simulink model "text28"  (R2014a)
settings: Solver=FixedStepDiscrete  StartTime=0.0  StopTime=10.0  FixedStep=0.0005  RelTol=1e-3
libraries: simulink x70, ec55xxlib x61
(part 1 of 3)
settings Model: Creator=HP  LastModifiedBy=30858
settings OptimizationCC: InlineParams=on  InlineInvariantSignals=on  RollThreshold=9  StateBitsets=on  DataBitsets=on  UseTempVars=on  ZeroExternalMemoryAtStartup=off  ZeroInternalMemoryAtStartup=off  EfficientFloat2IntCast=on  OptimizeModelRefInitCode=on  LifeSpan=1
settings DebuggingCC: InheritedTsInSrcMsg=none
settings HardwareCC: ProdLargestAtomicInteger=Long  ProdLargestAtomicFloat=Double  ProdIntDivRoundTo=Zero  ProdEndianess=BigEndian  ProdHWDeviceType=Freescale MPC5500
settings RTWCC: SystemTargetFile=ec55xx.tlc  MakeCommand=make_rtw optimized_fixed_point=1  GenerateMakefile=off  TemplateMakefile=ec55xx_lcc.tmf  PostCodeGenCommand=ec55xx_pst_s2(buildInfo)  Description=Target for EC55XX  GenerateReport=on  ProcessScript=ec55xx_make_rtw_hook  IncludeHyperlinkInReport=on  LaunchReport=on
settings CodeAppCC: IgnoreCustomStorageClasses=off
settings STFCustomTargetCC: ModelReferenceCompliant=off  ConcurrentExecutionCompliant=off  IncludeMdlTerminateFcn=off  GeneratePreprocessorConditionals=Use local settings  CombineOutputUpdateFcns=on  SuppressErrorStatus=on  ERTCustomFileBanners=on  SupportContinuousTime=off  SupportNonInlinedSFcns=off  MATLABClassNameForMDSCustomization=Simulink.SoftwareTarget.ERTCustomization  GRTInterface=off  SystemTargetFile=ec55xx.tlc
settings ERTTargetCC: GenerateSampleERTMain=off  ModelReferenceCompliant=off  IncludeMdlTerminateFcn=off  SuppressErrorStatus=on  GenerateASAP2=on  ERTSrcFileBannerTemplate=ec55xx_code_template.cgt  ERTHdrFileBannerTemplate=ec55xx_code_template.cgt  ERTDataSrcFileTemplate=ec55xx_code_template.cgt  ERTDataHdrFileTemplate=ec55xx_code_template.cgt  ERTCustomFileTemplate=ec55xx_file_process.tlc

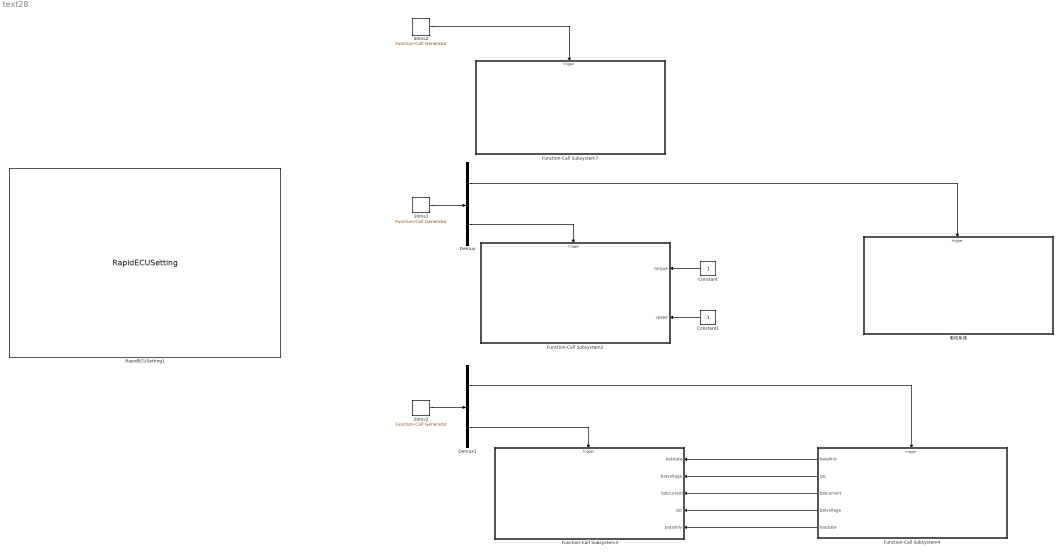
== system text28 ==
  10ms1 : simulink/Ports & Subsystems/Function-Call Generator  sample_time=0.01  numberOfIterations=1
  20ms2 : simulink/Ports & Subsystems/Function-Call Generator  sample_time=0.2  numberOfIterations=1
  50ms2 : simulink/Ports & Subsystems/Function-Call Generator  sample_time=0.05  numberOfIterations=1
  Constant : Constant
  Constant1 : Constant
  Demux : Demux  Outputs=2
  Demux1 : Demux  Outputs=2
  Function-Call Subsystem2 : Subsystem  TreatAsAtomicUnit=on
  Function-Call Subsystem3 : Subsystem  TreatAsAtomicUnit=on
  Function-Call Subsystem4 : Subsystem  TreatAsAtomicUnit=on
  Function-Call Subsystem7 : Subsystem  TreatAsAtomicUnit=on
  RapidECUSetting1 : ec55xxlib/RapidECU_U2/RapidECUSetting
      link override CAN: apdf=1  acmt=Extended(29-bit ID)  bcmt=Extended(29-bit ID)  ccmt=Standard(11-bit ID)
      link override CCP: idtype=Extended(29-bit ID)
      link override CPU: wdgenable=on  counter=104ms
      link override RTI: rtiperiod=0.0005
  驱动系统 : Subsystem  TreatAsAtomicUnit=on
  wires:
  10ms1/1 -> Demux/1
  20ms2/1 -> Demux1/1
  50ms2/1 -> Function-Call Subsystem7/Trigger
  Demux/1 -> 驱动系统/Trigger
  Demux/2 -> Function-Call Subsystem2/Trigger
  Demux1/1 -> Function-Call Subsystem4/Trigger
  Demux1/2 -> Function-Call Subsystem3/Trigger
  Function-Call Subsystem4/1(batalmlv) -> Function-Call Subsystem3/1(batstate)
  Function-Call Subsystem4/2(soc) -> Function-Call Subsystem3/2(batvoltage)
  Function-Call Subsystem4/3(batcurrent) -> Function-Call Subsystem3/3(batcurrent)
  Function-Call Subsystem4/4(batvoltage) -> Function-Call Subsystem3/4(soc)
  Function-Call Subsystem4/5(batstate) -> Function-Call Subsystem3/5(batalmlv)
  Constant/1 -> Function-Call Subsystem2/1(torque)
  Constant1/1 -> Function-Call Subsystem2/2(speed)

== system text28/Function-Call Subsystem2 ==
  torque : Inport
  speed : Inport  Port=2
  function : TriggerPort  TriggerType=function-call
  CANTransmit : ec55xxlib/RapidECU_U2/07CANCommucation/CANTransmit  canmodule=A  canbuffer=8  canmessageid=hex2dec('3E4')  canmessagetype=Standard(11-bit ID)  datalength=8  sampletime=-1
  xieyi : Subsystem
  xieyi_Ter : Terminator
  wires:
  CANTransmit/1 -> xieyi_Ter/1
  xieyi/1(output) -> CANTransmit/1
  speed/1 -> xieyi/1(Speed_in)
  torque/1 -> xieyi/2(Motor_toque_in)

== system text28/Function-Call Subsystem3 ==
  batstate : Inport
  batvoltage : Inport  Port=2
  batcurrent : Inport  Port=3
  soc : Inport  Port=4
  batalmlv : Inport  Port=5
  function : TriggerPort  TriggerType=function-call
  CANTransmit : ec55xxlib/RapidECU_U2/07CANCommucation/CANTransmit  canmodule=A  canbuffer=8  canmessageid=hex2dec('015')  canmessagetype=Standard(11-bit ID)  datalength=8  sampletime=-1
  dianchi : Subsystem
  dianchi_Ter : Terminator
  wires:
  CANTransmit/1 -> dianchi_Ter/1
  dianchi/1(output) -> CANTransmit/1
  batvoltage/1 -> dianchi/3(BatVoltage_in)
  batstate/1 -> dianchi/1(BatState_in)
  batalmlv/1 -> dianchi/2(BatAlmLv_in)
  soc/1 -> dianchi/4(BatSoc_in)
  batcurrent/1 -> dianchi/5(BatCurrent_in)

== system text28/Function-Call Subsystem4 ==
  function : TriggerPort  TriggerType=function-call
  CAN检测 : ec55xxlib/RapidECU_U2/07CANCommucation/CANReceive  canmodule=A  canbuffer=0  canmessageid=hex2dec('186040F3')  canmessagetype=Extended(29-bit ID)  datalength=8  sampletime=-1
  Function-Call Subsystem4 : Subsystem  TreatAsAtomicUnit=on
  Logical Operator : Logic  Inputs=3  AllPortsSameDT=off  OutDataTypeStr=boolean
  MeaModule2 : ec55xxlib/RapidECU_U2/11Calibration/MeaModule  signal=bms_sign
  MeaModule5 : ec55xxlib/RapidECU_U2/11Calibration/MeaModule  signal=bms_canok
  ReceiveMessages : Subsystem
  Terminator : Terminator
  Terminator1 : Terminator
  Terminator3 : Terminator
  "can断线 " : Subsystem
  一级警告 : Subsystem
  可视 : Subsystem
  故障状态报警 : Subsystem
  batalmlv : Outport
  soc : Outport  Port=2
  batcurrent : Outport  Port=3
  batvoltage : Outport  Port=4
  batstate : Outport  Port=5
  wires:
  CAN检测/1 -> Function-Call Subsystem4/Trigger
  CAN检测/5 -> Terminator1/1
  CAN检测/4 -> Function-Call Subsystem4/2(In3)
  MeaModule5/1 -> Function-Call Subsystem4/1(1n1)
  CAN检测/3 -> Terminator3/1
  ReceiveMessages/1(batstate) -> 故障状态报警/1(In1), batstate/1
  Logical Operator/1 -> MeaModule2/1
  一级警告/1(Out1) -> Logical Operator/2
  故障状态报警/1(Out1) -> Logical Operator/1
  CAN检测/2 -> "can断线 "/1(In1), MeaModule5/1
  Function-Call Subsystem4/1(Out1) -> ReceiveMessages/1(In1)
  ReceiveMessages/2("batalmlv ") -> 一级警告/1(In1), batalmlv/1
  ReceiveMessages/3(soc) -> soc/1
  ReceiveMessages/4(batcurrent) -> batcurrent/1
  ReceiveMessages/5(batvoltage) -> batvoltage/1
  "can断线 "/1(Out1) -> Logical Operator/3
  MeaModule2/1 -> Terminator/1

== system text28/Function-Call Subsystem7 ==
  function : TriggerPort  TriggerType=function-call
  Constant1 : Constant  Value=50
  Constant2 : Constant  Value=50
  Constant3 : Constant
  Data Type Conversion1 : DataTypeConversion  OutDataTypeStr=uint32
  Data Type Conversion2 : DataTypeConversion  OutDataTypeStr=uint32
  Function-Call Subsystem2 : Subsystem  TreatAsAtomicUnit=on
  Logical Operator : Logic  Operator=OR  AllPortsSameDT=off  OutDataTypeStr=boolean
  MCU STATUS 2 : ec55xxlib/RapidECU_U2/07CANCommucation/CANReceive  canmodule=B  canbuffer=0  canmessageid=hex2dec('CFF0109 ')  canmessagetype=Extended(29-bit ID)  datalength=8  sampletime=-1
  MCU_STATUS_2 : Subsystem
  MeaModule : ec55xxlib/RapidECU_U1/11Calibration/MeaModule  signal=FAN_sign
  PowerDriverPWM : ec55xxlib/RapidECU_U2/06PowerDriverPWM/PowerDriverPWM  channel=118: O_PWM12_HS2A9  sampletime=-1
  Relational Operator : RelationalOperator  OutDataTypeStr=boolean
  Relational Operator1 : RelationalOperator  OutDataTypeStr=boolean
  Terminator2 : Terminator
  Terminator4 : Terminator
  Terminator5 : Terminator
  wires:
  MCU STATUS 2/1 -> Function-Call Subsystem2/Trigger
  MCU STATUS 2/3 -> Terminator2/1
  MCU STATUS 2/5 -> Terminator4/1
  MCU STATUS 2/2 -> Terminator5/1
  Function-Call Subsystem2/1(out1) -> MCU_STATUS_2/1(In1)
  MCU STATUS 2/4 -> Function-Call Subsystem2/1(In1)
  MCU_STATUS_2/1(Motor_Tem) -> Relational Operator/1
  MCU_STATUS_2/2(MCU_Tem) -> Relational Operator1/1
  Relational Operator/1 -> Logical Operator/1
  Relational Operator1/1 -> Logical Operator/2
  Constant1/1 -> Relational Operator1/2
  Constant2/1 -> Relational Operator/2
  Data Type Conversion1/1 -> PowerDriverPWM/2
  Constant3/1 -> Data Type Conversion2/1
  Data Type Conversion2/1 -> PowerDriverPWM/1
  Logical Operator/1 -> MeaModule/1
  MeaModule/1 -> Data Type Conversion1/1

== system text28/驱动系统 ==
  function : TriggerPort  TriggerType=function-call
  Constant : Constant
  Data Type Conversion : DataTypeConversion  OutDataTypeStr=boolean
  ECU : Subsystem
  MCU_CAN发送 : Subsystem
  MainRelaySwitch : ec55xxlib/RapidECU_U2/09PowerManagement/MainRelaySwitch  sampletime=-1
  WDGFeed : ec55xxlib/RapidECU_U2/08MCUManagement/WDGFeed  sampletime=-1
  安全回路输出 : Subsystem
  驱动逻辑 : Subsystem
  wires:
  ECU/1(Out1) -> MCU_CAN发送/1(In1)
  Data Type Conversion/1 -> MainRelaySwitch/1
  驱动逻辑/2(复位) -> ECU/2(保留)
  驱动逻辑/1(油门输出) -> ECU/1(扭矩请求)
  Constant/1 -> Data Type Conversion/1
  MCU_CAN发送/1(系统关键信号) -> 安全回路输出/1(In1)
  驱动逻辑/4(系统关键信号) -> 安全回路输出/2(In2)
  驱动逻辑/3(使能) -> ECU/3(使能)
  ? -> ?
  ? -> ?
  ? -> ?
  ? -> ?

== system text28/Function-Call Subsystem2/xieyi ==
  Speed_in : Inport
  Motor_toque_in : Inport  Port=2
  Conv{1..8} (8 alike) : DataTypeConversion
  Motor_toque : Subsystem
  Speed : Subsystem
  or{1..8} (8 alike) : simulink/Logic and Bit Operations/Bitwise Operator  logicop=OR  UseBitMask=off  NumInputPorts=2  BitMask=bin2dec('11011001')  BitMaskRealWorld=Stored Integer
  xieyi_DLC : Constant  Value=2  OutDataTypeStr=uint8
  xieyi_DLC_Out : Terminator
  xieyi_ID : Constant  Value=995  OutDataTypeStr=single
  xieyi_ID_Out : Terminator
  xieyi_mux : Mux  Inputs=8
  output : Outport
  wires:
  xieyi_mux/1 -> output/1
  Speed/1(output1) -> or1/1
  Speed/2(output2) -> or2/1
  Speed/3(output3) -> or3/1
  Speed/4(output4) -> or4/1
  Speed/5(output5) -> or5/1
  Speed/6(output6) -> or6/1
  Speed/7(output7) -> or7/1
  Speed/8(output8) -> or8/1
  Motor_toque/1(output1) -> or1/2
  Motor_toque/2(output2) -> or2/2
  Motor_toque/3(output3) -> or3/2
  Motor_toque/4(output4) -> or4/2
  Motor_toque/5(output5) -> or5/2
  Motor_toque/6(output6) -> or6/2
  Motor_toque/7(output7) -> or7/2
  Motor_toque/8(output8) -> or8/2
  or1/1 -> Conv1/1
  Conv1/1 -> xieyi_mux/1
  or2/1 -> Conv2/1
  Conv2/1 -> xieyi_mux/2
  or3/1 -> Conv3/1
  Conv3/1 -> xieyi_mux/3
  or4/1 -> Conv4/1
  Conv4/1 -> xieyi_mux/4
  or5/1 -> Conv5/1
  Conv5/1 -> xieyi_mux/5
  or6/1 -> Conv6/1
  Conv6/1 -> xieyi_mux/6
  or7/1 -> Conv7/1
  Conv7/1 -> xieyi_mux/7
  or8/1 -> Conv8/1
  Conv8/1 -> xieyi_mux/8
  xieyi_ID/1 -> xieyi_ID_Out/1
  xieyi_DLC/1 -> xieyi_DLC_Out/1
  Speed_in/1 -> Speed/1(Speed)
  Motor_toque_in/1 -> Motor_toque/1(Motor_toque)

== system text28/Function-Call Subsystem3/dianchi ==
  BatState_in : Inport
  BatAlmLv_in : Inport  Port=2
  BatVoltage_in : Inport  Port=3
  BatSoc_in : Inport  Port=4
  BatCurrent_in : Inport  Port=5
  BatAlmLv : Subsystem
  BatCurrent : Subsystem
  BatSoc : Subsystem
  BatState : Subsystem
  BatVoltage : Subsystem
  Conv{1..8} (8 alike) : DataTypeConversion
  dianchi_DLC : Constant  Value=7  OutDataTypeStr=uint8
  dianchi_DLC_Out : Terminator
  dianchi_ID : Constant  Value=2556444915  OutDataTypeStr=single
  dianchi_ID_Out : Terminator
  dianchi_mux : Mux  Inputs=8
  or{1..8} (8 alike) : simulink/Logic and Bit Operations/Bitwise Operator  logicop=OR  UseBitMask=off  NumInputPorts=5  BitMask=bin2dec('11011001')  BitMaskRealWorld=Stored Integer
  output : Outport
  wires:
  dianchi_mux/1 -> output/1
  BatState/1(output1) -> or1/1
  BatState/2(output2) -> or2/1
  BatState/3(output3) -> or3/1
  BatState/4(output4) -> or4/1
  BatState/5(output5) -> or5/1
  BatState/6(output6) -> or6/1
  BatState/7(output7) -> or7/1
  BatState/8(output8) -> or8/1
  BatAlmLv/1(output1) -> or1/2
  BatAlmLv/2(output2) -> or2/2
  BatAlmLv/3(output3) -> or3/2
  BatAlmLv/4(output4) -> or4/2
  BatAlmLv/5(output5) -> or5/2
  BatAlmLv/6(output6) -> or6/2
  BatAlmLv/7(output7) -> or7/2
  BatAlmLv/8(output8) -> or8/2
  BatVoltage/1(output1) -> or1/3
  BatVoltage/2(output2) -> or2/3
  BatVoltage/3(output3) -> or3/3
  BatVoltage/4(output4) -> or4/3
  BatVoltage/5(output5) -> or5/3
  BatVoltage/6(output6) -> or6/3
  BatVoltage/7(output7) -> or7/3
  BatVoltage/8(output8) -> or8/3
  BatSoc/1(output1) -> or1/4
  BatSoc/2(output2) -> or2/4
  BatSoc/3(output3) -> or3/4
  BatSoc/4(output4) -> or4/4
  BatSoc/5(output5) -> or5/4
  BatSoc/6(output6) -> or6/4
  BatSoc/7(output7) -> or7/4
  BatSoc/8(output8) -> or8/4
  BatCurrent/1(output1) -> or1/5
  BatCurrent/2(output2) -> or2/5
  BatCurrent/3(output3) -> or3/5
  BatCurrent/4(output4) -> or4/5
  BatCurrent/5(output5) -> or5/5
  BatCurrent/6(output6) -> or6/5
  BatCurrent/7(output7) -> or7/5
  BatCurrent/8(output8) -> or8/5
  or1/1 -> Conv1/1
  Conv1/1 -> dianchi_mux/1
  or2/1 -> Conv2/1
  Conv2/1 -> dianchi_mux/2
  or3/1 -> Conv3/1
  Conv3/1 -> dianchi_mux/3
  or4/1 -> Conv4/1
  Conv4/1 -> dianchi_mux/4
  or5/1 -> Conv5/1
  Conv5/1 -> dianchi_mux/5
  or6/1 -> Conv6/1
  Conv6/1 -> dianchi_mux/6
  or7/1 -> Conv7/1
  Conv7/1 -> dianchi_mux/7
  or8/1 -> Conv8/1
  Conv8/1 -> dianchi_mux/8
  dianchi_ID/1 -> dianchi_ID_Out/1
  dianchi_DLC/1 -> dianchi_DLC_Out/1
  BatState_in/1 -> BatState/1(BatState)
  BatAlmLv_in/1 -> BatAlmLv/1(BatAlmLv)
  BatVoltage_in/1 -> BatVoltage/1(BatVoltage)
  BatSoc_in/1 -> BatSoc/1(BatSoc)
  BatCurrent_in/1 -> BatCurrent/1(BatCurrent)

== system text28/Function-Call Subsystem4/Function-Call Subsystem4 ==
  1n1 : Inport
  In3 : Inport  Port=2
  function : TriggerPort  TriggerType=function-call
  Terminator2 : Terminator
  Out1 : Outport
  wires:
  1n1/1 -> Terminator2/1
  In3/1 -> Out1/1

== system text28/Function-Call Subsystem4/ReceiveMessages ==
  In1 : Inport
  BMS_HCU_INFO : Subsystem
  BatLife_Ter : Terminator
  BtaSOH_Ter : Terminator
  MeaModule : ec55xxlib/RapidECU_U2/11Calibration/MeaModule  signal=baojing
  MeaModule1 : ec55xxlib/RapidECU_U2/11Calibration/MeaModule  signal=soc
  MeaModule2 : ec55xxlib/RapidECU_U2/11Calibration/MeaModule  signal=zhuangtai
  MeaModule3 : ec55xxlib/RapidECU_U2/11Calibration/MeaModule  signal=dianya
  batstate : Outport
  "batalmlv " : Outport  Port=2
  soc : Outport  Port=3
  batcurrent : Outport  Port=4
  batvoltage : Outport  Port=5
  wires:
  BMS_HCU_INFO/1(BtaSOH_Out) -> BtaSOH_Ter/1
  BMS_HCU_INFO/5(BatLife_Out) -> BatLife_Ter/1
  BMS_HCU_INFO/6(BatCurrent_Out) -> batcurrent/1
  In1/1 -> BMS_HCU_INFO/1(input)
  BMS_HCU_INFO/7(BatAlmLv_Out) -> MeaModule/1
  MeaModule/1 -> "batalmlv "/1
  BMS_HCU_INFO/4(BatSoc_Out) -> MeaModule1/1
  MeaModule1/1 -> soc/1
  BMS_HCU_INFO/3(BatState_Out) -> MeaModule2/1
  MeaModule2/1 -> batstate/1
  BMS_HCU_INFO/2(BatVoltage_Out) -> MeaModule3/1
  MeaModule3/1 -> batvoltage/1

== system text28/Function-Call Subsystem4/can断线  ==
  In1 : Inport
  If Action Subsystem2 : Subsystem  TreatAsAtomicUnit=on
  If Action Subsystem3 : Subsystem  TreatAsAtomicUnit=on
  If1 : If  IfExpression=u1<1
  MeaModule1 : ec55xxlib/RapidECU_U2/11Calibration/MeaModule  signal=bms_sign1
  Merge1 : Merge
  Out1 : Outport
  wires:
  If1/1 -> If Action Subsystem2/Action
  If Action Subsystem2/1(Out1) -> Merge1/1
  MeaModule1/1 -> Out1/1
  If1/2 -> If Action Subsystem3/Action
  If Action Subsystem3/1(Out1) -> Merge1/2
  Merge1/1 -> MeaModule1/1
  In1/1 -> If1/1

== system text28/Function-Call Subsystem4/一级警告 ==
  In1 : Inport
  If : If  IfExpression=u1==1
  If Action Subsystem : Subsystem  TreatAsAtomicUnit=on
  If Action Subsystem1 : Subsystem  TreatAsAtomicUnit=on
  Merge : Merge
  Out1 : Outport
  wires:
  If/1 -> If Action Subsystem/Action
  If/2 -> If Action Subsystem1/Action
  In1/1 -> If/1
  If Action Subsystem/1(Out1) -> Merge/1
  If Action Subsystem1/1(Out1) -> Merge/2
  Merge/1 -> Out1/1

== system text28/Function-Call Subsystem4/可视 ==
  Add : Sum  OutDataTypeStr=uint32
  Constant1 : Constant  OutDataTypeStr=uint32
  Constant4 : Constant  OutDataTypeStr=uint32  SampleTime=-1
  Constant5 : Constant  Value=0  OutDataTypeStr=uint32  SampleTime=-1
  Constant6 : Constant
  Data Type Conversion4 : DataTypeConversion
  Data Type Conversion5 : DataTypeConversion  OutDataTypeStr=uint32
  Display : Display
  Display1 : Display
  MeaModule3 : ec55xxlib/RapidECU_U2/11Calibration/MeaModule  signal=keshi
  Switch : Switch  Criteria=u2 > Threshold  Threshold=5
  Unit Delay : UnitDelay  SampleTime=-1
  断can线亮灯3 : ec55xxlib/RapidECU_U2/06PowerDriverPWM/PowerDriverPWM  channel=58: O_PWM1_LS1A8  sampletime=-1
  wires:
  Data Type Conversion5/1 -> 断can线亮灯3/1
  Data Type Conversion4/1 -> 断can线亮灯3/2
  MeaModule3/1 -> Display/1, Data Type Conversion4/1
  Constant6/1 -> Data Type Conversion5/1
  Constant1/1 -> Add/1
  Constant4/1 -> Switch/1
  Switch/1 -> MeaModule3/1
  Add/1 -> Unit Delay/1, Display1/1, Switch/2
  Unit Delay/1 -> Add/2
  Constant5/1 -> Switch/3

== system text28/Function-Call Subsystem4/故障状态报警 ==
  In1 : Inport
  If : If  IfExpression=u1==7
  If Action Subsystem : Subsystem  TreatAsAtomicUnit=on
  If Action Subsystem1 : Subsystem  TreatAsAtomicUnit=on
  Merge : Merge
  Out1 : Outport
  wires:
  If/1 -> If Action Subsystem/Action
  If/2 -> If Action Subsystem1/Action
  In1/1 -> If/1
  If Action Subsystem/1(Out1) -> Merge/1
  If Action Subsystem1/1(Out1) -> Merge/2
  Merge/1 -> Out1/1

== system text28/Function-Call Subsystem7/Function-Call Subsystem2 ==
  In1 : Inport
  function : TriggerPort  TriggerType=function-call
  out1 : Outport
  wires:
  In1/1 -> out1/1

== system text28/Function-Call Subsystem7/MCU_STATUS_2 ==
  In1 : Inport
  Fail_Grade_out : Terminator
  Live_counter_Ter : Terminator
  MCU_STATUS_2 : Subsystem
  MeaModule5 : ec55xxlib/RapidECU_U1/11Calibration/MeaModule  signal=MotorTemp
  MeaModule6 : ec55xxlib/RapidECU_U1/11Calibration/MeaModule  signal=McuTemp
  Torque_Limit_High_Ter : Terminator
  Torque_Limit_Low_Ter : Terminator
  Motor_Tem : Outport
  MCU_Tem : Outport  Port=2
  wires:
  MCU_STATUS_2/1(Torque_Limit_Low_Out) -> Torque_Limit_Low_Ter/1
  MCU_STATUS_2/2(Torque_Limit_High_Out) -> Torque_Limit_High_Ter/1
  MCU_STATUS_2/5(Live_counter_Out) -> Live_counter_Ter/1
  MCU_STATUS_2/6(Fail_Grade_Out) -> Fail_Grade_out/1
  In1/1 -> MCU_STATUS_2/1(input)
  MeaModule5/1 -> Motor_Tem/1
  MCU_STATUS_2/3(Motor_Temperature_Out) -> MeaModule5/1
  MeaModule6/1 -> MCU_Tem/1
  MCU_STATUS_2/4(MCU_temperature_Out) -> MeaModule6/1

== system text28/驱动系统/ECU ==
  扭矩请求 : Inport
  保留 : Inport  Port=2
  使能 : Inport  Port=3
  Constant : Constant  Value=2
  Constant1 : Constant
  Constant2 : Constant  Value=9000
  FootBrake : Ground
  demand_speed : Ground
  handBrake : Ground
  电机报文打包 : Subsystem
  Out1 : Outport
  wires:
  Constant/1 -> 电机报文打包/8(Control_Mode_in)
  FootBrake/1 -> 电机报文打包/6(FootBrake_in)
  handBrake/1 -> 电机报文打包/5(handBrake_in)
  电机报文打包/1(output) -> Out1/1
  Constant1/1 -> 电机报文打包/7(Gear_in)
  保留/1 -> 电机报文打包/9(Fault_Reset_in)
  使能/1 -> 电机报文打包/10(MCU_Enable_in)
  demand_speed/1 -> 电机报文打包/1(Demand_Speed_in)
  Constant2/1 -> 电机报文打包/4(High_Value_in), 电机报文打包/3(Low_Value_in)
  扭矩请求/1 -> 电机报文打包/2(Demand_Torquee_in)

== system text28/驱动系统/MCU_CAN发送 ==
  In1 : Inport
  CANTransmit : ec55xxlib/RapidECU_U2/07CANCommucation/CANTransmit  canmodule=B  canbuffer=8  canmessageid=hex2dec('CFF09EF')  canmessagetype=Extended(29-bit ID)  datalength=8  sampletime=-1
  MeaModule : ec55xxlib/RapidECU_U2/11Calibration/MeaModule  signal=CAN_ok
  Terminator : Terminator
  安全回路out : Subsystem
  系统关键信号 : Outport
  wires:
  CANTransmit/1 -> MeaModule/1
  In1/1 -> CANTransmit/1
  MeaModule/1 -> 安全回路out/1(CAN ok), Terminator/1
  安全回路out/1(Out1) -> 系统关键信号/1

== system text28/驱动系统/安全回路输出 ==
  In1 : Inport
  In2 : Inport  Port=2
  Constant4 : Constant  OutDataTypeStr=uint32
  Data Type Conversion2 : DataTypeConversion  OutDataTypeStr=uint32
  Logical Operator : Logic  AllPortsSameDT=off  OutDataTypeStr=boolean
  MeaModule1 : ec55xxlib/RapidECU_U2/11Calibration/MeaModule  signal=anquan_out
  安全出 : ec55xxlib/RapidECU_U2/06PowerDriverPWM/PowerDriverPWM  channel=114: O_PWM9_HS2A9  sampletime=-1
  wires:
  Data Type Conversion2/1 -> MeaModule1/1
  Constant4/1 -> 安全出/1
  MeaModule1/1 -> 安全出/2
  Logical Operator/1 -> Data Type Conversion2/1
  In1/1 -> Logical Operator/1
  In2/1 -> Logical Operator/2

== system text28/驱动系统/驱动逻辑 ==
  Drive_AEKF : Subsystem
  制动与尾灯 : Subsystem  TreatAsAtomicUnit=on
  制动与待驶 : Subsystem
  油门规则 : Subsystem
  电机测速 : Subsystem
  角度传感器 : Subsystem
  油门输出 : Outport
  复位 : Outport  Port=2
  使能 : Outport  Port=3
  系统关键信号 : Outport  Port=4
  wires:
  制动与待驶/2(EN) -> 使能/1
  制动与待驶/1(RES) -> 复位/1
  角度传感器/3(系统关键信号判断) -> 系统关键信号/1
  角度传感器/1("油门数值 ") -> 油门规则/1(油门原始值)
  角度传感器/2(油门百分比) -> 油门规则/2(油门百分比)
  电机测速/2(电机扭矩) -> Drive_AEKF/3(Te_raw)
  电机测速/1(电机转速) -> Drive_AEKF/2(w_rpm)
  制动与尾灯/1(油压2) -> 油门规则/3(刹车有效)
  制动与尾灯/2(油压1) -> 制动与待驶/1("制动 ")
  油门规则/1(油门请求) -> Drive_AEKF/1(T_base)
  Drive_AEKF/1(T_opt) -> 油门输出/1

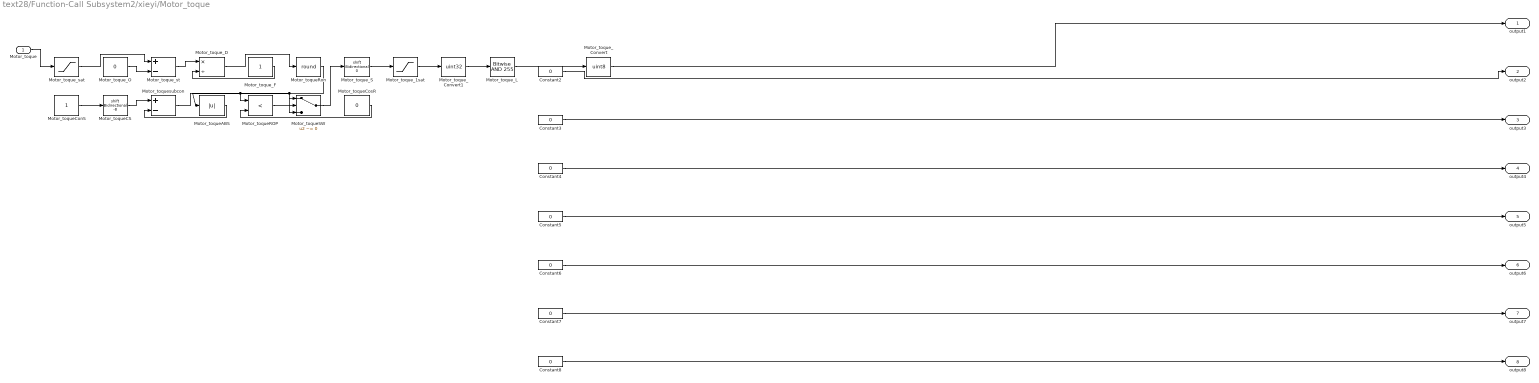
== system text28/Function-Call Subsystem2/xieyi/Motor_toque ==
  Motor_toque : Inport
  Constant{2..8} (7 alike) : Constant  Value=0  OutDataTypeStr=uint8  SampleTime=-1
  Motor_toqueABS : Abs
  Motor_toqueCS : ArithShift  BitShiftNumber=-8
  Motor_toqueConS : Constant  OutDataTypeStr=single
  Motor_toqueCosR : Constant  Value=0  OutDataTypeStr=uint8
  Motor_toqueROP : RelationalOperator  Operator=<  OutDataTypeStr=boolean
  Motor_toqueRon : Rounding  Operator=round
  Motor_toqueSW : Switch  Criteria=u2 ~= 0
  Motor_toque_1sat : Saturate  UpperLimit=255  LowerLimit=0
  Motor_toque_Convert : DataTypeConversion  OutDataTypeStr=uint8
  Motor_toque_Convert1 : DataTypeConversion  OutDataTypeStr=uint32
  Motor_toque_D : Product  Inputs=*/
  Motor_toque_F : Constant  OutDataTypeStr=single
  Motor_toque_L : simulink/Logic and Bit Operations/Bitwise Operator  logicop=AND  UseBitMask=on  BitMask=255  BitMaskRealWorld=Stored Integer
  Motor_toque_O : Constant  Value=0  OutDataTypeStr=single
  Motor_toque_S : ArithShift
  Motor_toque_sat : Saturate  UpperLimit=150  LowerLimit=0
  Motor_toque_st : Sum  Inputs=+-
  Motor_toquesubcon : Sum  Inputs=+-
  output1 : Outport
  output2 : Outport  Port=2
  output3 : Outport  Port=3
  output4 : Outport  Port=4
  output5 : Outport  Port=5
  output6 : Outport  Port=6
  output7 : Outport  Port=7
  output8 : Outport  Port=8
  wires:
  Motor_toque/1 -> Motor_toque_sat/1
  Motor_toque_sat/1 -> Motor_toque_st/1
  Motor_toque_O/1 -> Motor_toque_st/2
  Motor_toque_st/1 -> Motor_toque_D/1
  Motor_toque_F/1 -> Motor_toque_D/2
  Motor_toque_D/1 -> Motor_toqueRon/1
  Motor_toqueRon/1 -> Motor_toqueROP/1, Motor_toqueABS/1, Motor_toqueSW/3
  Motor_toqueCosR/1 -> Motor_toqueROP/2
  Motor_toqueConS/1 -> Motor_toqueCS/1
  Motor_toqueCS/1 -> Motor_toquesubcon/1
  Motor_toqueABS/1 -> Motor_toquesubcon/2
  Motor_toquesubcon/1 -> Motor_toqueSW/1
  Motor_toqueROP/1 -> Motor_toqueSW/2
  Motor_toqueSW/1 -> Motor_toque_S/1
  Motor_toque_S/1 -> Motor_toque_1sat/1
  Motor_toque_1sat/1 -> Motor_toque_Convert1/1
  Motor_toque_Convert1/1 -> Motor_toque_L/1
  Motor_toque_L/1 -> Motor_toque_Convert/1
  Motor_toque_Convert/1 -> output1/1
  Constant2/1 -> output2/1
  Constant3/1 -> output3/1
  Constant4/1 -> output4/1
  Constant5/1 -> output5/1
  Constant6/1 -> output6/1
  Constant7/1 -> output7/1
  Constant8/1 -> output8/1

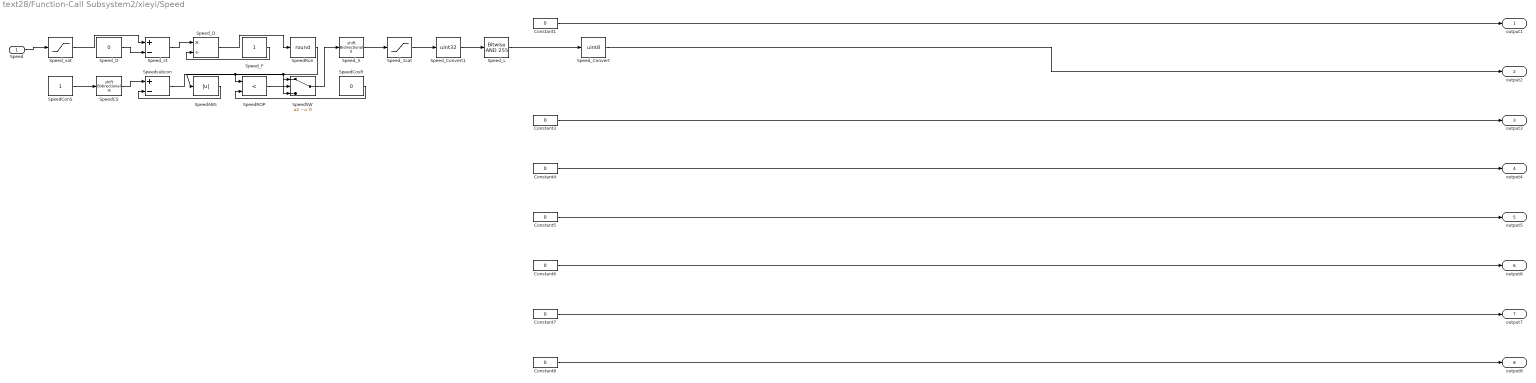
== system text28/Function-Call Subsystem2/xieyi/Speed ==
  Speed : Inport
  Constant{1,3..8} (7 alike) : Constant  Value=0  OutDataTypeStr=uint8  SampleTime=-1
  SpeedABS : Abs
  SpeedCS : ArithShift  BitShiftNumber=-8
  SpeedConS : Constant  OutDataTypeStr=single
  SpeedCosR : Constant  Value=0  OutDataTypeStr=uint8
  SpeedROP : RelationalOperator  Operator=<  OutDataTypeStr=boolean
  SpeedRon : Rounding  Operator=round
  SpeedSW : Switch  Criteria=u2 ~= 0
  Speed_1sat : Saturate  UpperLimit=255  LowerLimit=0
  Speed_Convert : DataTypeConversion  OutDataTypeStr=uint8
  Speed_Convert1 : DataTypeConversion  OutDataTypeStr=uint32
  Speed_D : Product  Inputs=*/
  Speed_F : Constant  OutDataTypeStr=single
  Speed_L : simulink/Logic and Bit Operations/Bitwise Operator  logicop=AND  UseBitMask=on  BitMask=255  BitMaskRealWorld=Stored Integer
  Speed_O : Constant  Value=0  OutDataTypeStr=single
  Speed_S : ArithShift
  Speed_sat : Saturate  UpperLimit=150  LowerLimit=0
  Speed_st : Sum  Inputs=+-
  Speedsubcon : Sum  Inputs=+-
  output1 : Outport
  output2 : Outport  Port=2
  output3 : Outport  Port=3
  output4 : Outport  Port=4
  output5 : Outport  Port=5
  output6 : Outport  Port=6
  output7 : Outport  Port=7
  output8 : Outport  Port=8
  wires:
  Speed/1 -> Speed_sat/1
  Speed_sat/1 -> Speed_st/1
  Speed_O/1 -> Speed_st/2
  Speed_st/1 -> Speed_D/1
  Speed_F/1 -> Speed_D/2
  Speed_D/1 -> SpeedRon/1
  SpeedRon/1 -> SpeedROP/1, SpeedABS/1, SpeedSW/3
  SpeedCosR/1 -> SpeedROP/2
  SpeedConS/1 -> SpeedCS/1
  SpeedCS/1 -> Speedsubcon/1
  SpeedABS/1 -> Speedsubcon/2
  Speedsubcon/1 -> SpeedSW/1
  SpeedROP/1 -> SpeedSW/2
  SpeedSW/1 -> Speed_S/1
  Speed_S/1 -> Speed_1sat/1
  Speed_1sat/1 -> Speed_Convert1/1
  Speed_Convert1/1 -> Speed_L/1
  Speed_L/1 -> Speed_Convert/1
  Speed_Convert/1 -> output2/1
  Constant1/1 -> output1/1
  Constant3/1 -> output3/1
  Constant4/1 -> output4/1
  Constant5/1 -> output5/1
  Constant6/1 -> output6/1
  Constant7/1 -> output7/1
  Constant8/1 -> output8/1

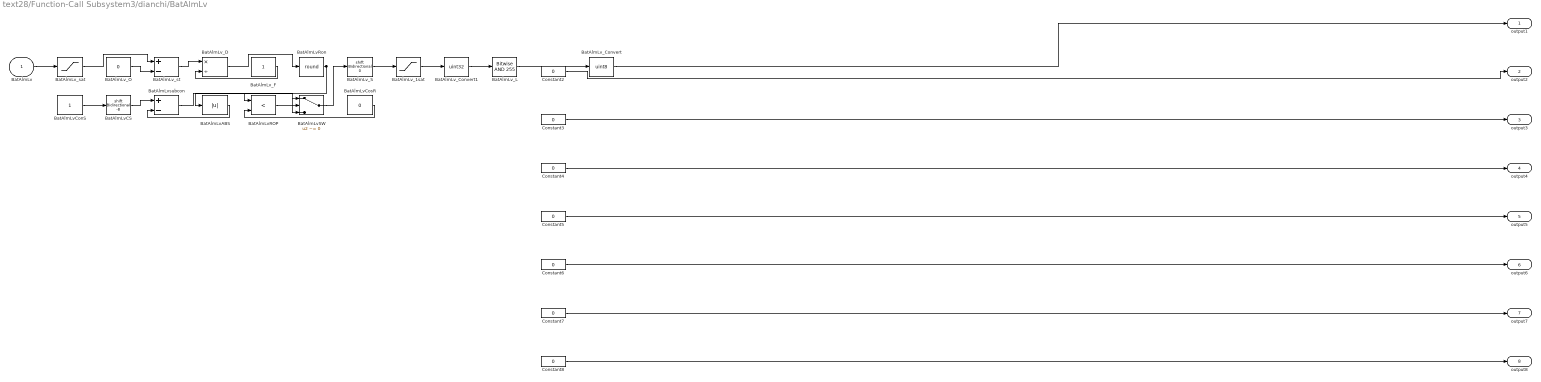
== system text28/Function-Call Subsystem3/dianchi/BatAlmLv ==
  BatAlmLv : Inport
  BatAlmLvABS : Abs
  BatAlmLvCS : ArithShift  BitShiftNumber=-8
  BatAlmLvConS : Constant  OutDataTypeStr=single
  BatAlmLvCosR : Constant  Value=0  OutDataTypeStr=uint8
  BatAlmLvROP : RelationalOperator  Operator=<  OutDataTypeStr=boolean
  BatAlmLvRon : Rounding  Operator=round
  BatAlmLvSW : Switch  Criteria=u2 ~= 0
  BatAlmLv_1sat : Saturate  UpperLimit=255  LowerLimit=0
  BatAlmLv_Convert : DataTypeConversion  OutDataTypeStr=uint8
  BatAlmLv_Convert1 : DataTypeConversion  OutDataTypeStr=uint32
  BatAlmLv_D : Product  Inputs=*/
  BatAlmLv_F : Constant  OutDataTypeStr=single
  BatAlmLv_L : simulink/Logic and Bit Operations/Bitwise Operator  logicop=AND  UseBitMask=on  BitMask=255  BitMaskRealWorld=Stored Integer
  BatAlmLv_O : Constant  Value=0  OutDataTypeStr=single
  BatAlmLv_S : ArithShift
  BatAlmLv_sat : Saturate  UpperLimit=4  LowerLimit=0
  BatAlmLv_st : Sum  Inputs=+-
  BatAlmLvsubcon : Sum  Inputs=+-
  Constant{2..8} (7 alike) : Constant  Value=0  OutDataTypeStr=uint8  SampleTime=-1
  output1 : Outport
  output2 : Outport  Port=2
  output3 : Outport  Port=3
  output4 : Outport  Port=4
  output5 : Outport  Port=5
  output6 : Outport  Port=6
  output7 : Outport  Port=7
  output8 : Outport  Port=8
  wires:
  BatAlmLv/1 -> BatAlmLv_sat/1
  BatAlmLv_sat/1 -> BatAlmLv_st/1
  BatAlmLv_O/1 -> BatAlmLv_st/2
  BatAlmLv_st/1 -> BatAlmLv_D/1
  BatAlmLv_F/1 -> BatAlmLv_D/2
  BatAlmLv_D/1 -> BatAlmLvRon/1
  BatAlmLvRon/1 -> BatAlmLvROP/1, BatAlmLvABS/1, BatAlmLvSW/3
  BatAlmLvCosR/1 -> BatAlmLvROP/2
  BatAlmLvConS/1 -> BatAlmLvCS/1
  BatAlmLvCS/1 -> BatAlmLvsubcon/1
  BatAlmLvABS/1 -> BatAlmLvsubcon/2
  BatAlmLvsubcon/1 -> BatAlmLvSW/1
  BatAlmLvROP/1 -> BatAlmLvSW/2
  BatAlmLvSW/1 -> BatAlmLv_S/1
  BatAlmLv_S/1 -> BatAlmLv_1sat/1
  BatAlmLv_1sat/1 -> BatAlmLv_Convert1/1
  BatAlmLv_Convert1/1 -> BatAlmLv_L/1
  BatAlmLv_L/1 -> BatAlmLv_Convert/1
  BatAlmLv_Convert/1 -> output1/1
  Constant2/1 -> output2/1
  Constant3/1 -> output3/1
  Constant4/1 -> output4/1
  Constant5/1 -> output5/1
  Constant6/1 -> output6/1
  Constant7/1 -> output7/1
  Constant8/1 -> output8/1

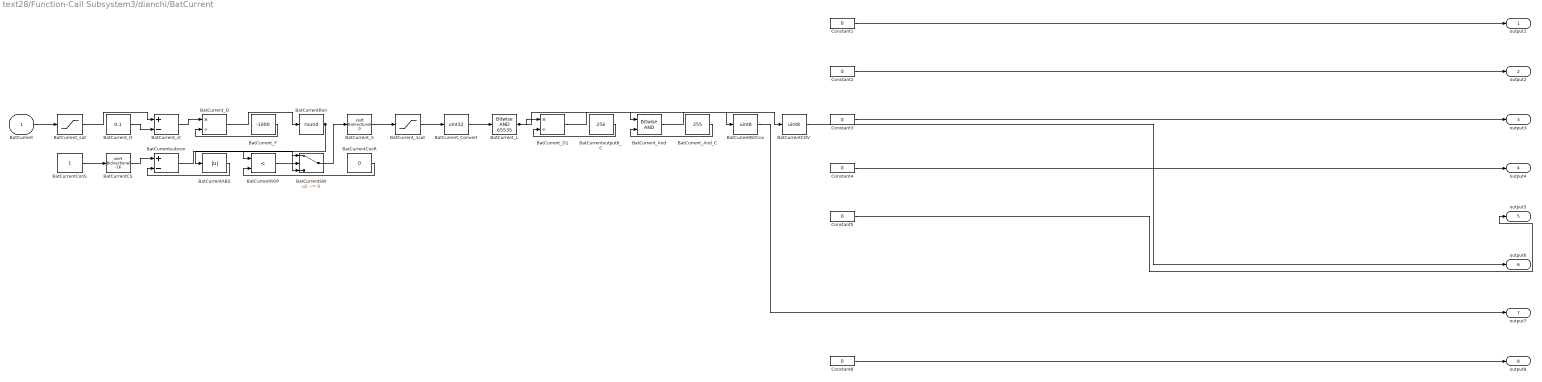
== system text28/Function-Call Subsystem3/dianchi/BatCurrent ==
  BatCurrent : Inport
  BatCurrentABS : Abs
  BatCurrentBitCov : DataTypeConversion  OutDataTypeStr=uint8
  BatCurrentCOV : DataTypeConversion  OutDataTypeStr=uint8
  BatCurrentCS : ArithShift  BitShiftNumber=-16
  BatCurrentConS : Constant  OutDataTypeStr=single
  BatCurrentCosR : Constant  Value=0  OutDataTypeStr=uint8
  BatCurrentROP : RelationalOperator  Operator=<  OutDataTypeStr=boolean
  BatCurrentRon : Rounding  Operator=round
  BatCurrentSW : Switch  Criteria=u2 ~= 0
  BatCurrent_1sat : Saturate  UpperLimit=65535  LowerLimit=0
  BatCurrent_And : simulink/Logic and Bit Operations/Bitwise Operator  logicop=AND  UseBitMask=off  NumInputPorts=2  BitMask=bin2dec('11011001')  BitMaskRealWorld=Stored Integer
  BatCurrent_And_C : Constant  Value=255  OutDataTypeStr=uint32
  BatCurrent_Convert : DataTypeConversion  OutDataTypeStr=uint32
  BatCurrent_D : Product  Inputs=*/
  BatCurrent_D1 : Product  Inputs=*/
  BatCurrent_F : Constant  Value=-1000  OutDataTypeStr=single
  BatCurrent_L : simulink/Logic and Bit Operations/Bitwise Operator  logicop=AND  UseBitMask=on  BitMask=65535  BitMaskRealWorld=Stored Integer
  BatCurrent_O : Constant  Value=0.1  OutDataTypeStr=single
  BatCurrent_S : ArithShift
  BatCurrent_sat : Saturate  UpperLimit=1000  LowerLimit=-1000
  BatCurrent_st : Sum  Inputs=+-
  BatCurrentoutput6_C : Constant  Value=256
  BatCurrentsubcon : Sum  Inputs=+-
  Constant{1..5,8} (6 alike) : Constant  Value=0  OutDataTypeStr=uint8  SampleTime=-1
  output1 : Outport
  output2 : Outport  Port=2
  output3 : Outport  Port=3
  output4 : Outport  Port=4
  output5 : Outport  Port=5
  output6 : Outport  Port=6
  output7 : Outport  Port=7
  output8 : Outport  Port=8
  wires:
  BatCurrent/1 -> BatCurrent_sat/1
  BatCurrent_sat/1 -> BatCurrent_st/1
  BatCurrent_O/1 -> BatCurrent_st/2
  BatCurrent_st/1 -> BatCurrent_D/1
  BatCurrent_F/1 -> BatCurrent_D/2
  BatCurrent_D/1 -> BatCurrentRon/1
  BatCurrentRon/1 -> BatCurrentROP/1, BatCurrentABS/1, BatCurrentSW/3
  BatCurrentCosR/1 -> BatCurrentROP/2
  BatCurrentConS/1 -> BatCurrentCS/1
  BatCurrentCS/1 -> BatCurrentsubcon/1
  BatCurrentABS/1 -> BatCurrentsubcon/2
  BatCurrentsubcon/1 -> BatCurrentSW/1
  BatCurrentROP/1 -> BatCurrentSW/2
  BatCurrentSW/1 -> BatCurrent_S/1
  BatCurrent_S/1 -> BatCurrent_1sat/1
  BatCurrent_1sat/1 -> BatCurrent_Convert/1
  BatCurrent_Convert/1 -> BatCurrent_L/1
  BatCurrent_L/1 -> BatCurrent_D1/1, BatCurrent_And/1
  BatCurrentoutput6_C/1 -> BatCurrent_D1/2
  BatCurrent_D1/1 -> BatCurrentCOV/1
  BatCurrentCOV/1 -> output6/1
  BatCurrent_And_C/1 -> BatCurrent_And/2
  BatCurrent_And/1 -> BatCurrentBitCov/1
  BatCurrentBitCov/1 -> output7/1
  Constant1/1 -> output1/1
  Constant2/1 -> output2/1
  Constant3/1 -> output3/1
  Constant4/1 -> output4/1
  Constant5/1 -> output5/1
  Constant8/1 -> output8/1

== system text28/Function-Call Subsystem3/dianchi/BatSoc ==
  BatSoc : Inport
  BatSocABS : Abs
  BatSocCS : ArithShift  BitShiftNumber=-8
  BatSocConS : Constant  OutDataTypeStr=single
  BatSocCosR : Constant  Value=0  OutDataTypeStr=uint8
  BatSocROP : RelationalOperator  Operator=<  OutDataTypeStr=boolean
  BatSocRon : Rounding  Operator=round
  BatSocSW : Switch  Criteria=u2 ~= 0
  BatSoc_1sat : Saturate  UpperLimit=255  LowerLimit=0
  BatSoc_Convert : DataTypeConversion  OutDataTypeStr=uint8
  BatSoc_Convert1 : DataTypeConversion  OutDataTypeStr=uint32
  BatSoc_D : Product  Inputs=*/
  BatSoc_F : Constant  OutDataTypeStr=single
  BatSoc_L : simulink/Logic and Bit Operations/Bitwise Operator  logicop=AND  UseBitMask=on  BitMask=255  BitMaskRealWorld=Stored Integer
  BatSoc_O : Constant  Value=0  OutDataTypeStr=single
  BatSoc_S : ArithShift
  BatSoc_sat : Saturate  UpperLimit=100  LowerLimit=0
  BatSoc_st : Sum  Inputs=+-
  BatSocsubcon : Sum  Inputs=+-
  Constant{1,3..8} (7 alike) : Constant  Value=0  OutDataTypeStr=uint8  SampleTime=-1
  output1 : Outport
  output2 : Outport  Port=2
  output3 : Outport  Port=3
  output4 : Outport  Port=4
  output5 : Outport  Port=5
  output6 : Outport  Port=6
  output7 : Outport  Port=7
  output8 : Outport  Port=8
  wires:
  BatSoc/1 -> BatSoc_sat/1
  BatSoc_sat/1 -> BatSoc_st/1
  BatSoc_O/1 -> BatSoc_st/2
  BatSoc_st/1 -> BatSoc_D/1
  BatSoc_F/1 -> BatSoc_D/2
  BatSoc_D/1 -> BatSocRon/1
  BatSocRon/1 -> BatSocROP/1, BatSocABS/1, BatSocSW/3
  BatSocCosR/1 -> BatSocROP/2
  BatSocConS/1 -> BatSocCS/1
  BatSocCS/1 -> BatSocsubcon/1
  BatSocABS/1 -> BatSocsubcon/2
  BatSocsubcon/1 -> BatSocSW/1
  BatSocROP/1 -> BatSocSW/2
  BatSocSW/1 -> BatSoc_S/1
  BatSoc_S/1 -> BatSoc_1sat/1
  BatSoc_1sat/1 -> BatSoc_Convert1/1
  BatSoc_Convert1/1 -> BatSoc_L/1
  BatSoc_L/1 -> BatSoc_Convert/1
  BatSoc_Convert/1 -> output2/1
  Constant1/1 -> output1/1
  Constant3/1 -> output3/1
  Constant4/1 -> output4/1
  Constant5/1 -> output5/1
  Constant6/1 -> output6/1
  Constant7/1 -> output7/1
  Constant8/1 -> output8/1

== system text28/Function-Call Subsystem3/dianchi/BatState ==
  BatState : Inport
  BatStateABS : Abs
  BatStateCS : ArithShift  BitShiftNumber=-8
  BatStateConS : Constant  OutDataTypeStr=single
  BatStateCosR : Constant  Value=0  OutDataTypeStr=uint8
  BatStateROP : RelationalOperator  Operator=<  OutDataTypeStr=boolean
  BatStateRon : Rounding  Operator=round
  BatStateSW : Switch  Criteria=u2 ~= 0
  BatState_1sat : Saturate  UpperLimit=255  LowerLimit=0
  BatState_Convert : DataTypeConversion  OutDataTypeStr=uint8
  BatState_Convert1 : DataTypeConversion  OutDataTypeStr=uint32
  BatState_D : Product  Inputs=*/
  BatState_F : Constant  OutDataTypeStr=single
  BatState_L : simulink/Logic and Bit Operations/Bitwise Operator  logicop=AND  UseBitMask=on  BitMask=255  BitMaskRealWorld=Stored Integer
  BatState_O : Constant  Value=0  OutDataTypeStr=single
  BatState_S : ArithShift
  BatState_sat : Saturate  UpperLimit=7  LowerLimit=1
  BatState_st : Sum  Inputs=+-
  BatStatesubcon : Sum  Inputs=+-
  Constant{1..2,4..8} (7 alike) : Constant  Value=0  OutDataTypeStr=uint8  SampleTime=-1
  output1 : Outport
  output2 : Outport  Port=2
  output3 : Outport  Port=3
  output4 : Outport  Port=4
  output5 : Outport  Port=5
  output6 : Outport  Port=6
  output7 : Outport  Port=7
  output8 : Outport  Port=8
  wires:
  BatState/1 -> BatState_sat/1
  BatState_sat/1 -> BatState_st/1
  BatState_O/1 -> BatState_st/2
  BatState_st/1 -> BatState_D/1
  BatState_F/1 -> BatState_D/2
  BatState_D/1 -> BatStateRon/1
  BatStateRon/1 -> BatStateROP/1, BatStateABS/1, BatStateSW/3
  BatStateCosR/1 -> BatStateROP/2
  BatStateConS/1 -> BatStateCS/1
  BatStateCS/1 -> BatStatesubcon/1
  BatStateABS/1 -> BatStatesubcon/2
  BatStatesubcon/1 -> BatStateSW/1
  BatStateROP/1 -> BatStateSW/2
  BatStateSW/1 -> BatState_S/1
  BatState_S/1 -> BatState_1sat/1
  BatState_1sat/1 -> BatState_Convert1/1
  BatState_Convert1/1 -> BatState_L/1
  BatState_L/1 -> BatState_Convert/1
  BatState_Convert/1 -> output3/1
  Constant1/1 -> output1/1
  Constant2/1 -> output2/1
  Constant4/1 -> output4/1
  Constant5/1 -> output5/1
  Constant6/1 -> output6/1
  Constant7/1 -> output7/1
  Constant8/1 -> output8/1

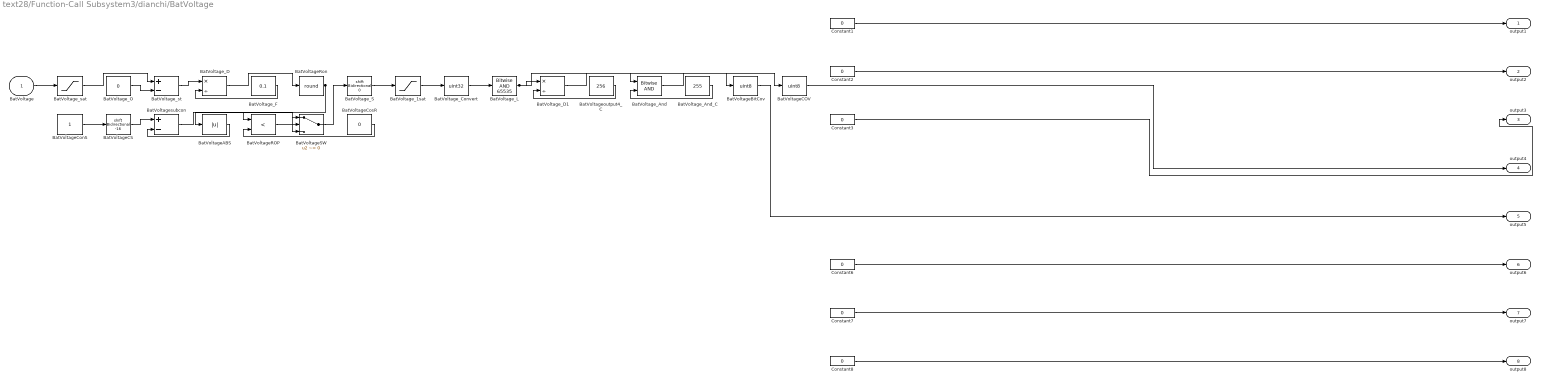
== system text28/Function-Call Subsystem3/dianchi/BatVoltage ==
  BatVoltage : Inport
  BatVoltageABS : Abs
  BatVoltageBitCov : DataTypeConversion  OutDataTypeStr=uint8
  BatVoltageCOV : DataTypeConversion  OutDataTypeStr=uint8
  BatVoltageCS : ArithShift  BitShiftNumber=-16
  BatVoltageConS : Constant  OutDataTypeStr=single
  BatVoltageCosR : Constant  Value=0  OutDataTypeStr=uint8
  BatVoltageROP : RelationalOperator  Operator=<  OutDataTypeStr=boolean
  BatVoltageRon : Rounding  Operator=round
  BatVoltageSW : Switch  Criteria=u2 ~= 0
  BatVoltage_1sat : Saturate  UpperLimit=65535  LowerLimit=0
  BatVoltage_And : simulink/Logic and Bit Operations/Bitwise Operator  logicop=AND  UseBitMask=off  NumInputPorts=2  BitMask=bin2dec('11011001')  BitMaskRealWorld=Stored Integer
  BatVoltage_And_C : Constant  Value=255  OutDataTypeStr=uint32
  BatVoltage_Convert : DataTypeConversion  OutDataTypeStr=uint32
  BatVoltage_D : Product  Inputs=*/
  BatVoltage_D1 : Product  Inputs=*/
  BatVoltage_F : Constant  Value=0.1  OutDataTypeStr=single
  BatVoltage_L : simulink/Logic and Bit Operations/Bitwise Operator  logicop=AND  UseBitMask=on  BitMask=65535  BitMaskRealWorld=Stored Integer
  BatVoltage_O : Constant  Value=0  OutDataTypeStr=single
  BatVoltage_S : ArithShift
  BatVoltage_sat : Saturate  UpperLimit=900  LowerLimit=0
  BatVoltage_st : Sum  Inputs=+-
  BatVoltageoutput4_C : Constant  Value=256
  BatVoltagesubcon : Sum  Inputs=+-
  Constant{1..3,6..8} (6 alike) : Constant  Value=0  OutDataTypeStr=uint8  SampleTime=-1
  output1 : Outport
  output2 : Outport  Port=2
  output3 : Outport  Port=3
  output4 : Outport  Port=4
  output5 : Outport  Port=5
  output6 : Outport  Port=6
  output7 : Outport  Port=7
  output8 : Outport  Port=8
  wires:
  BatVoltage/1 -> BatVoltage_sat/1
  BatVoltage_sat/1 -> BatVoltage_st/1
  BatVoltage_O/1 -> BatVoltage_st/2
  BatVoltage_st/1 -> BatVoltage_D/1
  BatVoltage_F/1 -> BatVoltage_D/2
  BatVoltage_D/1 -> BatVoltageRon/1
  BatVoltageRon/1 -> BatVoltageROP/1, BatVoltageABS/1, BatVoltageSW/3
  BatVoltageCosR/1 -> BatVoltageROP/2
  BatVoltageConS/1 -> BatVoltageCS/1
  BatVoltageCS/1 -> BatVoltagesubcon/1
  BatVoltageABS/1 -> BatVoltagesubcon/2
  BatVoltagesubcon/1 -> BatVoltageSW/1
  BatVoltageROP/1 -> BatVoltageSW/2
  BatVoltageSW/1 -> BatVoltage_S/1
  BatVoltage_S/1 -> BatVoltage_1sat/1
  BatVoltage_1sat/1 -> BatVoltage_Convert/1
  BatVoltage_Convert/1 -> BatVoltage_L/1
  BatVoltage_L/1 -> BatVoltage_D1/1, BatVoltage_And/1
  BatVoltageoutput4_C/1 -> BatVoltage_D1/2
  BatVoltage_D1/1 -> BatVoltageCOV/1
  BatVoltageCOV/1 -> output4/1
  BatVoltage_And_C/1 -> BatVoltage_And/2
  BatVoltage_And/1 -> BatVoltageBitCov/1
  BatVoltageBitCov/1 -> output5/1
  Constant1/1 -> output1/1
  Constant2/1 -> output2/1
  Constant3/1 -> output3/1
  Constant6/1 -> output6/1
  Constant7/1 -> output7/1
  Constant8/1 -> output8/1

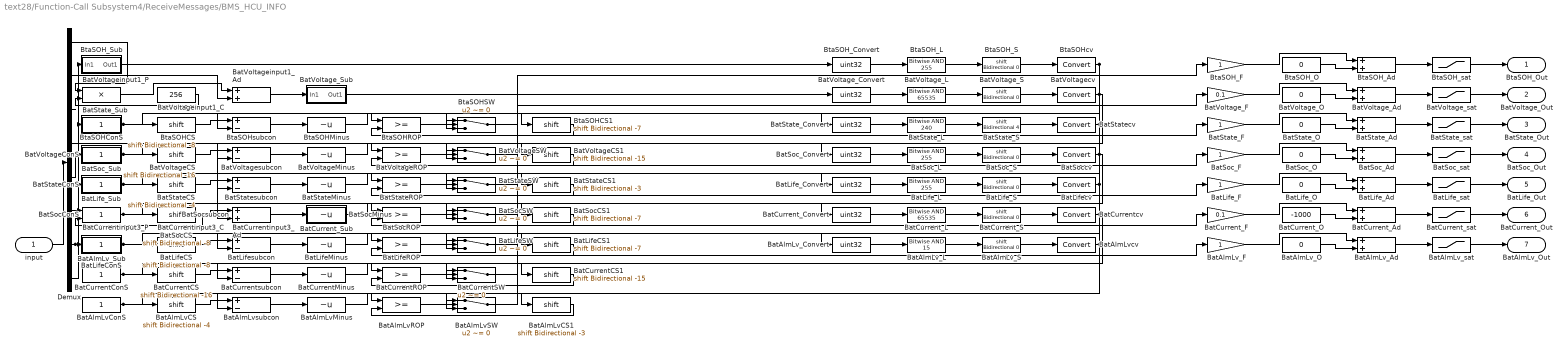
== system text28/Function-Call Subsystem4/ReceiveMessages/BMS_HCU_INFO ==
  input : Inport
  BatAlmLvCS : ArithShift  BitShiftNumber=-4
  BatAlmLvCS1 : ArithShift  BitShiftNumber=-3
  BatAlmLvConS : Constant  OutDataTypeStr=single
  BatAlmLvMinus : UnaryMinus
  BatAlmLvROP : RelationalOperator  OutDataTypeStr=boolean
  BatAlmLvSW : Switch  Criteria=u2 ~= 0
  BatAlmLv_Ad : Sum
  BatAlmLv_Convert : DataTypeConversion  OutDataTypeStr=uint32
  BatAlmLv_F : Gain
  BatAlmLv_L : simulink/Logic and Bit Operations/Bitwise Operator  logicop=AND  UseBitMask=on  BitMask=15  BitMaskRealWorld=Stored Integer
  BatAlmLv_O : Constant  Value=0  OutDataTypeStr=single
  BatAlmLv_S : ArithShift
  BatAlmLv_Sub : Subsystem
  BatAlmLv_sat : Saturate  UpperLimit=4  LowerLimit=0
  BatAlmLvcv : DataTypeConversion
  BatAlmLvsubcon : Sum  Inputs=+-
  BatCurrentCS : ArithShift  BitShiftNumber=-16
  BatCurrentCS1 : ArithShift  BitShiftNumber=-15
  BatCurrentConS : Constant  OutDataTypeStr=single
  BatCurrentMinus : UnaryMinus
  BatCurrentROP : RelationalOperator  OutDataTypeStr=boolean
  BatCurrentSW : Switch  Criteria=u2 ~= 0
  BatCurrent_Ad : Sum
  BatCurrent_Convert : DataTypeConversion  OutDataTypeStr=uint32
  BatCurrent_F : Gain  Gain=0.1
  BatCurrent_L : simulink/Logic and Bit Operations/Bitwise Operator  logicop=AND  UseBitMask=on  BitMask=65535  BitMaskRealWorld=Stored Integer
  BatCurrent_O : Constant  Value=-1000  OutDataTypeStr=single
  BatCurrent_S : ArithShift
  BatCurrent_Sub : Subsystem
  BatCurrent_sat : Saturate  UpperLimit=1000  LowerLimit=-1000
  BatCurrentcv : DataTypeConversion
  BatCurrentinput3_Ad : Sum
  BatCurrentinput3_C : Constant  Value=256
  BatCurrentinput3_P : Product
  BatCurrentsubcon : Sum  Inputs=+-
  BatLifeCS : ArithShift  BitShiftNumber=-8
  BatLifeCS1 : ArithShift  BitShiftNumber=-7
  BatLifeConS : Constant  OutDataTypeStr=single
  BatLifeMinus : UnaryMinus
  BatLifeROP : RelationalOperator  OutDataTypeStr=boolean
  BatLifeSW : Switch  Criteria=u2 ~= 0
  BatLife_Ad : Sum
  BatLife_Convert : DataTypeConversion  OutDataTypeStr=uint32
  BatLife_F : Gain
  BatLife_L : simulink/Logic and Bit Operations/Bitwise Operator  logicop=AND  UseBitMask=on  BitMask=255  BitMaskRealWorld=Stored Integer
  BatLife_O : Constant  Value=0  OutDataTypeStr=single
  BatLife_S : ArithShift
  BatLife_Sub : Subsystem
  BatLife_sat : Saturate  UpperLimit=255  LowerLimit=0
  BatLifecv : DataTypeConversion
  BatLifesubcon : Sum  Inputs=+-
  BatSocCS : ArithShift  BitShiftNumber=-8
  BatSocCS1 : ArithShift  BitShiftNumber=-7
  BatSocConS : Constant  OutDataTypeStr=single
  BatSocMinus : UnaryMinus
  BatSocROP : RelationalOperator  OutDataTypeStr=boolean
  BatSocSW : Switch  Criteria=u2 ~= 0
  BatSoc_Ad : Sum
  BatSoc_Convert : DataTypeConversion  OutDataTypeStr=uint32
  BatSoc_F : Gain
  BatSoc_L : simulink/Logic and Bit Operations/Bitwise Operator  logicop=AND  UseBitMask=on  BitMask=255  BitMaskRealWorld=Stored Integer
  BatSoc_O : Constant  Value=0  OutDataTypeStr=single
  BatSoc_S : ArithShift
  BatSoc_Sub : Subsystem
  BatSoc_sat : Saturate  UpperLimit=100  LowerLimit=0
  BatSoccv : DataTypeConversion
  BatSocsubcon : Sum  Inputs=+-
  BatStateCS : ArithShift  BitShiftNumber=-4
  BatStateCS1 : ArithShift  BitShiftNumber=-3
  BatStateConS : Constant  OutDataTypeStr=single
  BatStateMinus : UnaryMinus
  BatStateROP : RelationalOperator  OutDataTypeStr=boolean
  BatStateSW : Switch  Criteria=u2 ~= 0
  BatState_Ad : Sum
  BatState_Convert : DataTypeConversion  OutDataTypeStr=uint32
  BatState_F : Gain
  BatState_L : simulink/Logic and Bit Operations/Bitwise Operator  logicop=AND  UseBitMask=on  BitMask=240  BitMaskRealWorld=Stored Integer
  BatState_O : Constant  Value=0  OutDataTypeStr=single
  BatState_S : ArithShift  BitShiftNumber=4
  BatState_Sub : Subsystem
  BatState_sat : Saturate  UpperLimit=7  LowerLimit=1
  BatStatecv : DataTypeConversion
  BatStatesubcon : Sum  Inputs=+-
  BatVoltageCS : ArithShift  BitShiftNumber=-16
  BatVoltageCS1 : ArithShift  BitShiftNumber=-15
  BatVoltageConS : Constant  OutDataTypeStr=single
  BatVoltageMinus : UnaryMinus
  BatVoltageROP : RelationalOperator  OutDataTypeStr=boolean
  BatVoltageSW : Switch  Criteria=u2 ~= 0
  BatVoltage_Ad : Sum
  BatVoltage_Convert : DataTypeConversion  OutDataTypeStr=uint32
  BatVoltage_F : Gain  Gain=0.1
  BatVoltage_L : simulink/Logic and Bit Operations/Bitwise Operator  logicop=AND  UseBitMask=on  BitMask=65535  BitMaskRealWorld=Stored Integer
  BatVoltage_O : Constant  Value=0  OutDataTypeStr=single
  BatVoltage_S : ArithShift
  BatVoltage_Sub : Subsystem
  BatVoltage_sat : Saturate  UpperLimit=900  LowerLimit=0
  BatVoltagecv : DataTypeConversion
  BatVoltageinput1_Ad : Sum
  BatVoltageinput1_C : Constant  Value=256
  BatVoltageinput1_P : Product
  BatVoltagesubcon : Sum  Inputs=+-
  BtaSOHCS : ArithShift  BitShiftNumber=-8
  BtaSOHCS1 : ArithShift  BitShiftNumber=-7
  BtaSOHConS : Constant  OutDataTypeStr=single
  BtaSOHMinus : UnaryMinus
  BtaSOHROP : RelationalOperator  OutDataTypeStr=boolean
  BtaSOHSW : Switch  Criteria=u2 ~= 0
  BtaSOH_Ad : Sum
  BtaSOH_Convert : DataTypeConversion  OutDataTypeStr=uint32
  BtaSOH_F : Gain
  BtaSOH_L : simulink/Logic and Bit Operations/Bitwise Operator  logicop=AND  UseBitMask=on  BitMask=255  BitMaskRealWorld=Stored Integer
  BtaSOH_O : Constant  Value=0  OutDataTypeStr=single
  BtaSOH_S : ArithShift
  BtaSOH_Sub : Subsystem
  BtaSOH_sat : Saturate  UpperLimit=100  LowerLimit=0
  BtaSOHcv : DataTypeConversion
  BtaSOHsubcon : Sum  Inputs=+-
  Demux : Demux  Outputs=8
  BtaSOH_Out : Outport
  BatVoltage_Out : Outport  Port=2
  BatState_Out : Outport  Port=3
  BatSoc_Out : Outport  Port=4
  BatLife_Out : Outport  Port=5
  BatCurrent_Out : Outport  Port=6
  BatAlmLv_Out : Outport  Port=7
  wires:
  BtaSOH_F/1 -> BtaSOH_Ad/1
  BtaSOH_O/1 -> BtaSOH_Ad/2
  BtaSOH_Ad/1 -> BtaSOH_sat/1
  BtaSOH_sat/1 -> BtaSOH_Out/1
  Demux/6 -> BtaSOH_Sub/1(In1)
  BtaSOH_Sub/1(Out1) -> BtaSOH_Convert/1
  BtaSOH_Convert/1 -> BtaSOH_L/1
  BtaSOH_L/1 -> BtaSOH_S/1
  BtaSOH_S/1 -> BtaSOHcv/1
  BtaSOHcv/1 -> BtaSOHROP/1, BtaSOHsubcon/2, BtaSOHSW/3
  BtaSOHConS/1 -> BtaSOHCS/1, BtaSOHCS1/1
  BtaSOHCS1/1 -> BtaSOHROP/2
  BtaSOHCS/1 -> BtaSOHsubcon/1
  BtaSOHsubcon/1 -> BtaSOHMinus/1
  BtaSOHMinus/1 -> BtaSOHSW/1
  BtaSOHSW/1 -> BtaSOH_F/1
  BtaSOHROP/1 -> BtaSOHSW/2
  BatVoltage_F/1 -> BatVoltage_Ad/1
  BatVoltage_O/1 -> BatVoltage_Ad/2
  BatVoltage_Ad/1 -> BatVoltage_sat/1
  BatVoltage_sat/1 -> BatVoltage_Out/1
  Demux/1 -> BatVoltageinput1_P/1
  BatVoltageinput1_C/1 -> BatVoltageinput1_P/2
  BatVoltageinput1_P/1 -> BatVoltageinput1_Ad/1
  Demux/2 -> BatVoltageinput1_Ad/2
  BatVoltageinput1_Ad/1 -> BatVoltage_Sub/1(In1)
  BatVoltage_Sub/1(Out1) -> BatVoltage_Convert/1
  BatVoltage_Convert/1 -> BatVoltage_L/1
  BatVoltage_L/1 -> BatVoltage_S/1
  BatVoltage_S/1 -> BatVoltagecv/1
  BatVoltagecv/1 -> BatVoltageROP/1, BatVoltagesubcon/2, BatVoltageSW/3
  BatVoltageConS/1 -> BatVoltageCS/1, BatVoltageCS1/1
  BatVoltageCS1/1 -> BatVoltageROP/2
  BatVoltageCS/1 -> BatVoltagesubcon/1
  BatVoltagesubcon/1 -> BatVoltageMinus/1
  BatVoltageMinus/1 -> BatVoltageSW/1
  BatVoltageSW/1 -> BatVoltage_F/1
  BatVoltageROP/1 -> BatVoltageSW/2
  BatState_F/1 -> BatState_Ad/1
  BatState_O/1 -> BatState_Ad/2
  BatState_Ad/1 -> BatState_sat/1
  BatState_sat/1 -> BatState_Out/1
  Demux/7 -> BatState_Sub/1(In1), BatAlmLv_Sub/1(In1)
  BatState_Sub/1(Out1) -> BatState_Convert/1
  BatState_Convert/1 -> BatState_L/1
  BatState_L/1 -> BatState_S/1
  BatState_S/1 -> BatStatecv/1
  BatStatecv/1 -> BatStateROP/1, BatStatesubcon/2, BatStateSW/3
  BatStateConS/1 -> BatStateCS/1, BatStateCS1/1
  BatStateCS1/1 -> BatStateROP/2
  BatStateCS/1 -> BatStatesubcon/1
  BatStatesubcon/1 -> BatStateMinus/1
  BatStateMinus/1 -> BatStateSW/1
  BatStateSW/1 -> BatState_F/1
  BatStateROP/1 -> BatStateSW/2
  BatSoc_F/1 -> BatSoc_Ad/1
  BatSoc_O/1 -> BatSoc_Ad/2
  BatSoc_Ad/1 -> BatSoc_sat/1
  BatSoc_sat/1 -> BatSoc_Out/1
  Demux/5 -> BatSoc_Sub/1(In1)
  BatSoc_Sub/1(Out1) -> BatSoc_Convert/1
  BatSoc_Convert/1 -> BatSoc_L/1
  BatSoc_L/1 -> BatSoc_S/1
  BatSoc_S/1 -> BatSoccv/1
  BatSoccv/1 -> BatSocROP/1, BatSocsubcon/2, BatSocSW/3
  BatSocConS/1 -> BatSocCS/1, BatSocCS1/1
  BatSocCS1/1 -> BatSocROP/2
  BatSocCS/1 -> BatSocsubcon/1
  BatSocsubcon/1 -> BatSocMinus/1
  BatSocMinus/1 -> BatSocSW/1
  BatSocSW/1 -> BatSoc_F/1
  BatSocROP/1 -> BatSocSW/2
  BatLife_F/1 -> BatLife_Ad/1
  BatLife_O/1 -> BatLife_Ad/2
  BatLife_Ad/1 -> BatLife_sat/1
  BatLife_sat/1 -> BatLife_Out/1
  Demux/8 -> BatLife_Sub/1(In1)
  BatLife_Sub/1(Out1) -> BatLife_Convert/1
  BatLife_Convert/1 -> BatLife_L/1
  BatLife_L/1 -> BatLife_S/1
  BatLife_S/1 -> BatLifecv/1
  BatLifecv/1 -> BatLifeROP/1, BatLifesubcon/2, BatLifeSW/3
  BatLifeConS/1 -> BatLifeCS/1, BatLifeCS1/1
  BatLifeCS1/1 -> BatLifeROP/2
  BatLifeCS/1 -> BatLifesubcon/1
  BatLifesubcon/1 -> BatLifeMinus/1
  BatLifeMinus/1 -> BatLifeSW/1
  BatLifeSW/1 -> BatLife_F/1
  BatLifeROP/1 -> BatLifeSW/2
  BatCurrent_F/1 -> BatCurrent_Ad/1
  BatCurrent_O/1 -> BatCurrent_Ad/2
  BatCurrent_Ad/1 -> BatCurrent_sat/1
  BatCurrent_sat/1 -> BatCurrent_Out/1
  Demux/3 -> BatCurrentinput3_P/1
  BatCurrentinput3_C/1 -> BatCurrentinput3_P/2
  BatCurrentinput3_P/1 -> BatCurrentinput3_Ad/1
  Demux/4 -> BatCurrentinput3_Ad/2
  BatCurrentinput3_Ad/1 -> BatCurrent_Sub/1(In1)
  BatCurrent_Sub/1(Out1) -> BatCurrent_Convert/1
  BatCurrent_Convert/1 -> BatCurrent_L/1
  BatCurrent_L/1 -> BatCurrent_S/1
  BatCurrent_S/1 -> BatCurrentcv/1
  BatCurrentcv/1 -> BatCurrentROP/1, BatCurrentsubcon/2, BatCurrentSW/3
  BatCurrentConS/1 -> BatCurrentCS/1, BatCurrentCS1/1
  BatCurrentCS1/1 -> BatCurrentROP/2
  BatCurrentCS/1 -> BatCurrentsubcon/1
  BatCurrentsubcon/1 -> BatCurrentMinus/1
  BatCurrentMinus/1 -> BatCurrentSW/1
  BatCurrentSW/1 -> BatCurrent_F/1
  BatCurrentROP/1 -> BatCurrentSW/2
  BatAlmLv_F/1 -> BatAlmLv_Ad/1
  BatAlmLv_O/1 -> BatAlmLv_Ad/2
  BatAlmLv_Ad/1 -> BatAlmLv_sat/1
  BatAlmLv_sat/1 -> BatAlmLv_Out/1
  BatAlmLv_Sub/1(Out1) -> BatAlmLv_Convert/1
  BatAlmLv_Convert/1 -> BatAlmLv_L/1
  BatAlmLv_L/1 -> BatAlmLv_S/1
  BatAlmLv_S/1 -> BatAlmLvcv/1
  BatAlmLvcv/1 -> BatAlmLvROP/1, BatAlmLvsubcon/2, BatAlmLvSW/3
  BatAlmLvConS/1 -> BatAlmLvCS/1, BatAlmLvCS1/1
  BatAlmLvCS1/1 -> BatAlmLvROP/2
  BatAlmLvCS/1 -> BatAlmLvsubcon/1
  BatAlmLvsubcon/1 -> BatAlmLvMinus/1
  BatAlmLvMinus/1 -> BatAlmLvSW/1
  BatAlmLvSW/1 -> BatAlmLv_F/1
  BatAlmLvROP/1 -> BatAlmLvSW/2
  input/1 -> Demux/1

== system text28/Function-Call Subsystem4/can断线 /If Action Subsystem2 ==
  Action Port : ActionPort  ActionType=then
  Constant2 : Constant  Value=0
  Out1 : Outport
  wires:
  Constant2/1 -> Out1/1

== system text28/Function-Call Subsystem4/can断线 /If Action Subsystem3 ==
  Action Port : ActionPort  ActionType=else
  Constant2 : Constant
  Out1 : Outport
  wires:
  Constant2/1 -> Out1/1

== system text28/Function-Call Subsystem4/一级警告/If Action Subsystem ==
  Action Port : ActionPort  ActionType=then
  Constant : Constant  Value=0
  Out1 : Outport
  wires:
  Constant/1 -> Out1/1

== system text28/Function-Call Subsystem4/一级警告/If Action Subsystem1 ==
  Action Port : ActionPort  ActionType=else
  Constant : Constant
  Out1 : Outport
  wires:
  Constant/1 -> Out1/1

== system text28/Function-Call Subsystem4/故障状态报警/If Action Subsystem ==
  Action Port : ActionPort  ActionType=then
  Constant : Constant  Value=0
  Out1 : Outport
  wires:
  Constant/1 -> Out1/1

== system text28/Function-Call Subsystem4/故障状态报警/If Action Subsystem1 ==
  Action Port : ActionPort  ActionType=else
  Constant : Constant
  Out1 : Outport
  wires:
  Constant/1 -> Out1/1
